simulink subsystem "HMC5883L"  (R2021a)
settings: Solver=VariableStepAuto  StartTime=0.0  StopTime=10.0  RelTol=1e-3
undefined symbols (not defined in the file): mag
libraries: simulink x4
settings Model: Creator=jmher  LastModifiedBy=Laura

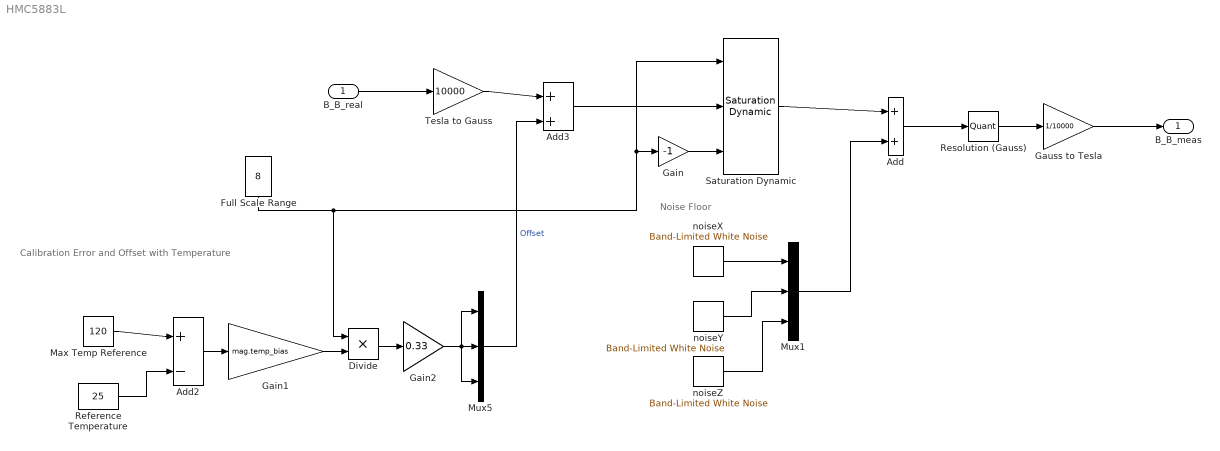
== system HMC5883L ==
  note: Noise Floor
  note: Calibration Error and Offset
      | with Temperature
  B_B_real : Inport
  Add : Sum  Inputs=+|+
  Add2 : Sum  Inputs=+|-
  Add3 : Sum  Inputs=+|+
  Divide : Product  Inputs=**
  Full Scale Range : Constant  Value=8
  Gain : Gain  Gain=-1
  Gain1 : Gain  Gain=mag.temp_bias
  Gain2 : Gain  Gain=0.33
  Gauss to Tesla : Gain  Gain=1/10000
  Max Temp Reference : Constant  Value=120
  Mux1 : Mux  Inputs=3
  Mux5 : Mux  Inputs=3
  Reference Temperature : Constant  Value=25
  Resolution (Gauss) : Quantizer  QuantizationInterval=mag.quantization  LinearizeAsGain=off
  Saturation Dynamic : simulink/Discontinuities/Saturation Dynamic  OutMin=[]  OutMax=[]  OutDataTypeStr=Inherit: Same as second input  OutDataType=fixdt(1, 16)  OutScaling=2^-10  RndMeth=Round  DoSatur=off
  Tesla to Gauss : Gain  Gain=10000
  noiseX : simulink/Sources/Band-Limited White Noise  Cov=mag.power_noise(1)  Ts=1/40  seed=[47561]
  noiseY : simulink/Sources/Band-Limited White Noise  Cov=mag.power_noise(2)  Ts=1/40  seed=[238641]
  noiseZ : simulink/Sources/Band-Limited White Noise  Cov=mag.power_noise(3)  Ts=1/40  seed=[23341]
  B_B_meas : Outport  SampleTime=1/10
  wires:
  Full Scale Range/1 -> Divide/1, Gain/1, Saturation Dynamic/1
  Gain/1 -> Saturation Dynamic/3
  noiseX/1 -> Mux1/1
  noiseY/1 -> Mux1/2
  noiseZ/1 -> Mux1/3
  Add/1 -> Resolution (Gauss)/1
  Mux1/1 -> Add/2
  Add2/1 -> Gain1/1
  Max Temp Reference/1 -> Add2/1
  Reference Temperature/1 -> Add2/2
  Add3/1 -> Saturation Dynamic/2
  Gain2/1 -> Mux5/2, Mux5/3, Mux5/1
  Mux5/1 -> Add3/2  "Offset"
  B_B_real/1 -> Tesla to Gauss/1
  Tesla to Gauss/1 -> Add3/1
  Divide/1 -> Gain2/1
  Gain1/1 -> Divide/2
  Saturation Dynamic/1 -> Add/1
  Resolution (Gauss)/1 -> Gauss to Tesla/1
  Gauss to Tesla/1 -> B_B_meas/1
